simulink model "PID"  (R2023b)
settings: Solver=VariableStepAuto  StartTime=0.0  StopTime=2  RelTol=1e-3
settings Model: Creator=satya  LastModifiedBy=satya
settings SolverCC: ZeroCrossAlgorithm=Adaptive
settings DebuggingCC: IgnoredZcDiagnostic=none

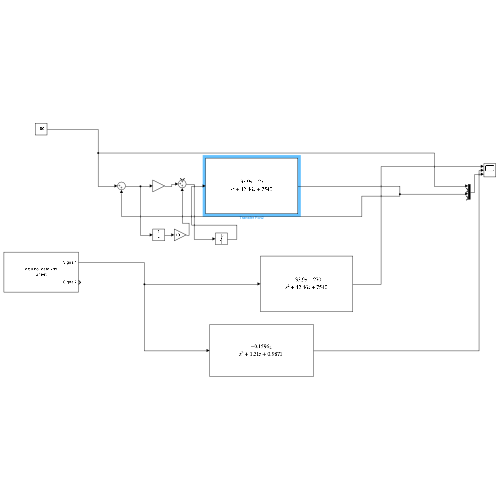
[thumbnail: Simulink's stored preview of the top-level diagram]
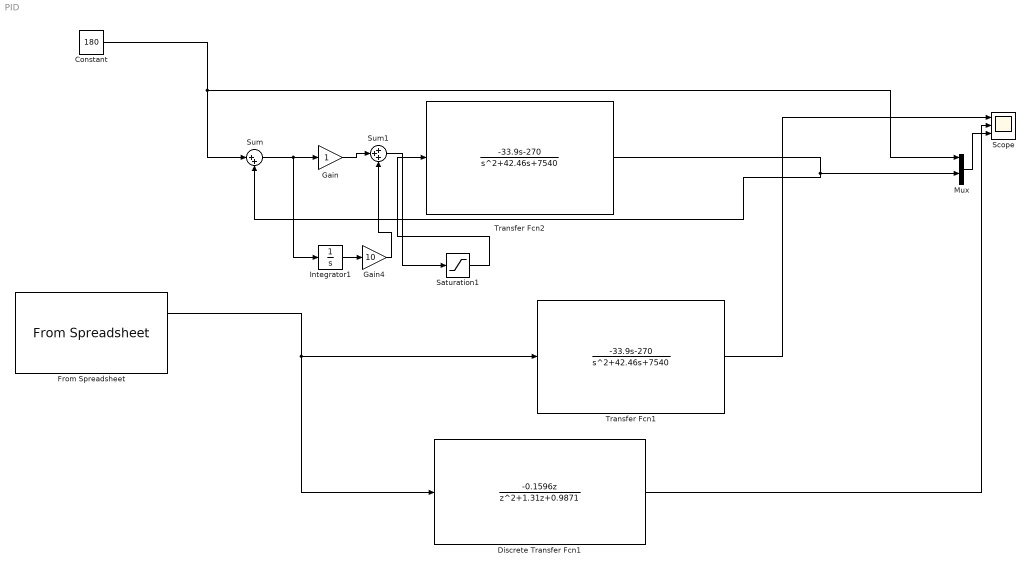
== system PID ==
  Constant : Constant  Value=180
  Discrete Transfer Fcn1 : DiscreteTransferFcn  Numerator=[ -0.1596 0]  Denominator=[1 1.31 0.9871]  InitialStates=1
  From Spreadsheet : FromSpreadsheet  FileName=arduino_data.xlsx  SheetName=Sheet  TreatFirstColumnAs=Data  SampleTime=0.002
  Gain : Gain
  Gain4 : Gain  Gain=10
  Integrator1 : Integrator
  Mux : Mux
  Saturation1 : Saturate  UpperLimit=255  LowerLimit=0
  Scope : Scope  NumInputPorts=3
  Sum : Sum  Inputs=|++
  Sum1 : Sum  Inputs=+++
  Transfer Fcn1 : TransferFcn  Numerator=[-33.9 -270 ]  Denominator=[1 42.46 7540]
  Transfer Fcn2 : TransferFcn  Numerator=[-33.9 -270 ]  Denominator=[1 42.46 7540]
  wires:
  Transfer Fcn2/1 -> Sum/2, Mux/3
  From Spreadsheet/1 -> Transfer Fcn1/1, Discrete Transfer Fcn1/1
  Gain/1 -> Sum1/2
  Sum/1 -> Integrator1/1, Gain/1
  Mux/1 -> Scope/3
  Sum1/1 -> Saturation1/1
  Saturation1/1 -> Transfer Fcn2/1
  Integrator1/1 -> Gain4/1
  Gain4/1 -> Sum1/3
  Constant/1 -> Sum/1, Mux/1
  Discrete Transfer Fcn1/1 -> Scope/2
  Transfer Fcn1/1 -> Scope/1
